simulink model "PD_con_G"  (R2024b)
settings: Solver=ode3  StartTime=0.0  StopTime=tsamplesimulink  FixedStep=0.001  MaxStep=0.001  RelTol=1e-3  AbsTol=1e-3  EnableMultiTasking=on
values from neighbouring files (symbols this model uses):
  Ac = [  0,       1,                 0,              0 ... (first row only)    [iniciar_backstepping_corregido.m]    (also in iniciar_elastico.m = [      0              1                         0           )
  Bcg = [  0,  0,              0,  Ka*Km/Jm ... (first row only)    [iniciar_backstepping_corregido.m]    (also in iniciar_elastico.m = [      0              0)
  Cc = [  eye(4) ... (first row only)    [iniciar_backstepping_corregido.m]    (also in iniciar_elastico.m = [      eye(4))
  Dcg = zeros(5,2)    [iniciar_backstepping_corregido.m]    (also in iniciar_elastico.m)
  g = 9.81    [iniciar_backstepping_corregido.m]    (also in iniciar_elastico.m)
  Ka = 0.18    [iniciar_backstepping_corregido.m]    (also in iniciar_elastico.m)
  Km = 0.11    [iniciar_backstepping_corregido.m]    (also in iniciar_elastico.m)
  Kp = 50    [iniciar_backstepping_corregido.m]    (also in iniciar_elastico.m = 80)
  Kv = 10    [iniciar_backstepping_corregido.m]    (also in iniciar_elastico.m = 160)
  m = size(obj, 1)    [expandir_entorno.m]    (also in iniciar_backstepping_corregido.m = 1; iniciar_elastico.m = 1; untitled5.m = (pi + pj)/2; verificar_Cfree.m = size(poligono, 1))
  N = size(matriz_costes,1)    [Dijkstra.m]    (also in Evitar_obstaculos.m = length (M); Ordenar_ptos.m = size(lista_puntos,1); dib_rectas.m = size(rectas,1); dib_rectas2.m = size(rectas,1))
  xc = 0.2    [iniciar_backstepping_corregido.m]    (also in iniciar_elastico.m)
settings Model: Creator=rzotovic  LastModifiedBy=ruizh
settings SolverCC: AutoScaleAbsTol=off  AlgebraicLoopSolver=TrustRegion
settings DataIOCC: SaveFormat=Array  SignalLoggingSaveFormat=ModelDataLogs  SaveOutput=off  SaveTime=off  ReturnWorkspaceOutputs=off
settings OptimizationCC: BlockReduction=off  BooleanDataType=off  ExpressionDepthLimit=2147483647  LifeSpan=inf
settings DebuggingCC: SaveWithParameterizedLinksMsg=none  UnderspecifiedInitializationDetection=Classic  MergeDetectMultiDrivingBlocksExec=none  SignalResolutionControl=TryResolveAllWithWarning  MultiTaskDSMMsg=warning  MultiTaskCondExecSysMsg=none  FcnCallInpInsideContextMsg=warning  UnconnectedInputMsg=warning  UnconnectedOutputMsg=warning  UnconnectedLineMsg=warning  StateNameClashWarn=warning  SFUnexpectedBacktrackingDiag=warning  SFNoUnconditionalDefaultTransitionDiag=warning  SFExecutionAtInitializationDiag=none  ArithmeticOperatorsInVariantConditions=warning
settings HardwareCC: ProdBitPerPointer=32  ProdBitPerSizeT=32  ProdBitPerPtrDiffT=32  ProdLargestAtomicFloat=None  ProdIntDivRoundTo=Undefined  ProdEndianess=Unspecified  ProdWordSize=32  ProdHWDeviceType=32-bit Generic  TargetUnknown=on
settings ModelReferenceCC: EnableRefExpFcnMdlSchedulingChecks=on  PropagateSignalLabelsOutOfModel=off
settings SFSimCC: SimUseLocalCustomCode=off  CustomCodeUndefinedFunction=UseInterfaceOnly
settings RTWCC: RTWUseLocalCustomCode=off  GPUComputeCapability=3.5
settings CodeAppCC: StateflowObjectComments=on
settings GRTTargetCC: TargetLangStandard=C89/C90 (ANSI)  CombineOutputUpdateFcns=off  GRTInterface=on
settings ConfigComp: CovMetricSettings=dw  CovSaveCumulativeToWorkspaceVar=on  CovSaveSingleToWorkspaceVar=on  CovExternalEMLEnable=off  CovSFcnEnable=off

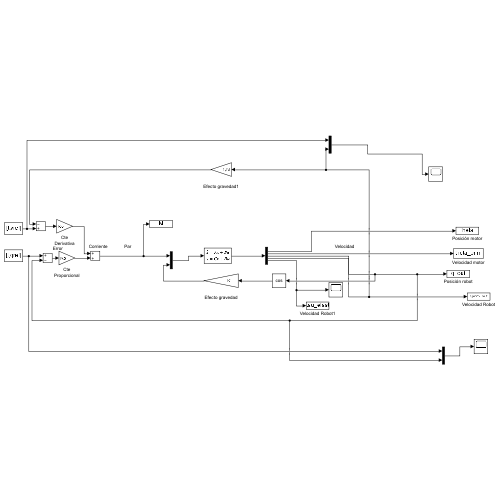
[thumbnail: Simulink's stored preview of the top-level diagram]
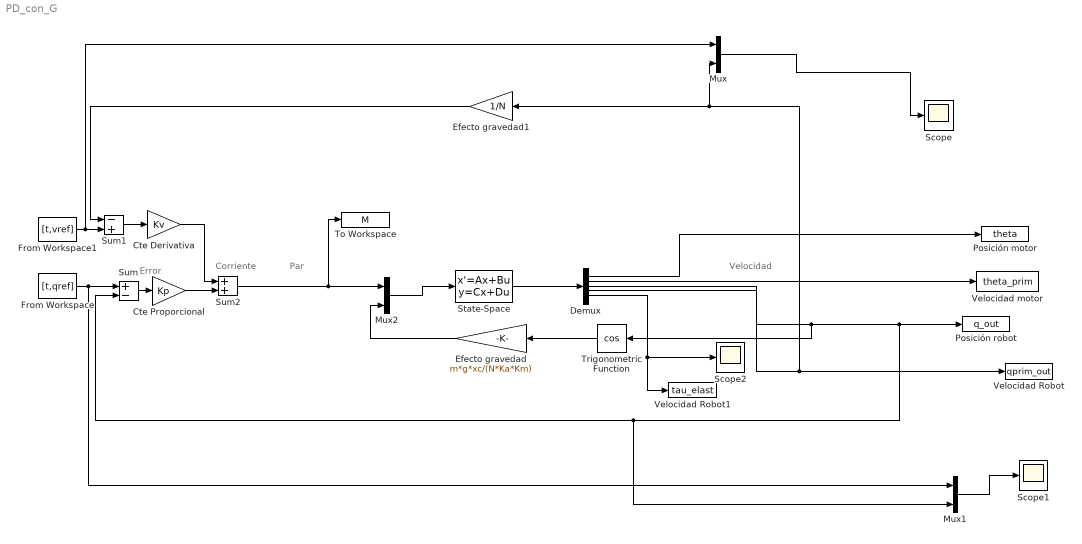
== system PD_con_G ==
  note: Corriente
  note: Par
  note: Velocidad
  note: Error
  " Efecto gravedad" : Gain  Gain=m*g*xc/(N*Ka*Km)  SaturateOnIntegerOverflow=on  OutDataTypeStr=Inherit: Same as input  ParamDataTypeStr=Inherit: Same as input
  " Efecto gravedad1" : Gain  Gain=1/N  SaturateOnIntegerOverflow=on  OutDataTypeStr=Inherit: Same as input  ParamDataTypeStr=Inherit: Same as input
  Cte Derivativa : Gain  Gain=Kv  SaturateOnIntegerOverflow=on  OutDataTypeStr=Inherit: Same as input  ParamDataTypeStr=Inherit: Same as input
  Cte Proporcional : Gain  Gain=Kp  SaturateOnIntegerOverflow=on  OutDataTypeStr=Inherit: Same as input  ParamDataTypeStr=Inherit: Same as input
  Demux : Demux  Outputs=5
  From Workspace : FromWorkspace  VariableName=[t,qref]  SampleTime=0.001  ZeroCross=off
  From Workspace1 : FromWorkspace  VariableName=[t,vref]  SampleTime=0.001  ZeroCross=off
  Mux : Mux  Inputs=2
  Mux1 : Mux  Inputs=2
  Mux2 : Mux  Inputs=2
  Posición motor : ToWorkspace  VariableName=theta
      settings: MaxDataPoints=samplesimulink
  Posición robot : ToWorkspace  VariableName=q_out
      settings: MaxDataPoints=samplesimulink
  Scope : Scope
  Scope1 : Scope
  Scope2 : Scope
  State-Space : StateSpace  A=Ac  B=Bcg  C=Cc  D=Dcg  InitialCondition=0
  Sum : Sum  Inputs=+-  InputSameDT=on  SaturateOnIntegerOverflow=on  OutDataTypeStr=Inherit: Same as first input
  Sum1 : Sum  Inputs=-+  InputSameDT=on  SaturateOnIntegerOverflow=on  OutDataTypeStr=Inherit: Same as first input
  Sum2 : Sum  InputSameDT=on  SaturateOnIntegerOverflow=on  OutDataTypeStr=Inherit: Same as first input
  To Workspace : ToWorkspace  VariableName=M
      settings: MaxDataPoints=11333
  Trigonometric Function : Trigonometry  Operator=cos
  Velocidad Robot : ToWorkspace  VariableName=qprim_out
      settings: MaxDataPoints=samplesimulink
  Velocidad Robot1 : ToWorkspace  VariableName=tau_elast
      settings: MaxDataPoints=samplesimulink
  Velocidad motor : ToWorkspace  VariableName=theta_prim
      settings: MaxDataPoints=samplesimulink
  wires:
  Sum/1 -> Cte Proporcional/1
  Sum1/1 -> Cte Derivativa/1
  From Workspace1/1 -> Mux/1, Sum1/2
  Cte Proporcional/1 -> Sum2/2
  Cte Derivativa/1 -> Sum2/1
  State-Space/1 -> Demux/1
  Demux/1 -> Posición motor/1
  Demux/2 -> Velocidad motor/1
  Demux/4 -> " Efecto gravedad1"/1, Mux/2, Velocidad Robot/1
  Mux/1 -> Scope/1
  Mux1/1 -> Scope1/1
  Demux/3 -> Trigonometric Function/1, Mux1/2, Sum/2, Posición robot/1
  From Workspace/1 -> Mux1/1, Sum/1
  Sum2/1 -> To Workspace/1, Mux2/1
  Mux2/1 -> State-Space/1
  Demux/5 -> Scope2/1, Velocidad Robot1/1
  Trigonometric Function/1 -> " Efecto gravedad"/1
  " Efecto gravedad"/1 -> Mux2/2
  " Efecto gravedad1"/1 -> Sum1/1
